simulink model "magSim3"  (Simulink 3.00)
settings: Solver=ode45  StartTime=0  StopTime=100  RelTol=1e-5
values from neighbouring files (symbols this model uses):
  Bmag = sscanf(get(findobj(gcf, 'Tag', 'EditTextBmag'),'String'), '    [CUBESIM bak.m]    (also in CUBESIM.m = sscanf(get(findobj(FIG, 'Tag', 'EditTextBmag'),'String'), '; current.mat = 1.28; current_bak.mat = 1.28; default.mat = 1.28)
  Br = 0.35    [CUBESIM bak.m]    (also in CUBESIM.m; current.mat; current_bak.mat; default.mat)
  Bs1 = sscanf(get(findobj(gcf, 'Tag', 'EditTextBs1'),'String'), '    [CUBESIM bak.m]    (also in CUBESIM.m = sscanf(get(findobj(FIG, 'Tag', 'EditTextBs1'),'String'), '; current.mat = 0.73; current_bak.mat = 0.73; default.mat = 0.73)
  Bs2 = sscanf(get(findobj(gcf, 'Tag', 'EditTextBs2'),'String'), '    [CUBESIM bak.m]    (also in CUBESIM.m = sscanf(get(findobj(FIG, 'Tag', 'EditTextBs2'),'String'), '; current.mat = 0.73; current_bak.mat = 0.73; default.mat = 0.73)
  fs = get(findobj(gcf, 'Tag', 'EditTextfs'),'UserData')    [CUBESIM bak.m]    (also in CUBESIM.m = get(findobj(FIG, 'Tag', 'EditTextfs'),'UserData'); current.mat = 0.0809149305556; current_bak.mat = 0.323659722222; default.mat = 0.161829861111)
  H0 = Isc * wb0    [CUBESIM bak.m]    (also in CUBESIM.m; current.mat = [0.00110737714815 0.0010993416399 0.00032293142175]; current_bak.mat = [-5e-05 -5e-05 0.001]; default.mat = [0 0 0.001])
  Hc = 1.59    [CUBESIM bak.m]    (also in CUBESIM.m; current.mat; current_bak.mat; default.mat = 1)
  Jinv = Isc^(-1)    [CUBESIM bak.m]    (also in CUBESIM.m; current.mat = [94.7867649385  0.000760150942758  0.106731312353; 0.0007601; current_bak.mat = [502.645502646  26.455026455  26.455026455; 26.455026455  50; default.mat = [500  0  0; 0  500  0; 0  0  500])
  q0 = [q1; q2; q3; q4]./sqrt(q1^2+q2^2+q3^2+q4^2)    [CUBESIM bak.m]    (also in CUBESIM.m; current.mat = [0 0 0 1]; current_bak.mat = [0 0 0 1]; default.mat = [0 0 0 1])
  sw = get(findobj(gcf, 'Tag', 'ButtonSW1'),'UserData')    [CUBESIM bak.m]    (also in CUBESIM.m = get(findobj(FIG, 'Tag', 'ButtonSW1'),'UserData'); current.mat = 1; current_bak.mat = 1; default.mat = 1)
  uhyst1 = [uhyst1x; uhyst1y; uhyst1z]./ norm([uhyst1x; uhyst1y; uhyst1z])    [CUBESIM bak.m]    (also in CUBESIM.m; current.mat = [0 1 0]; current_bak.mat = [0 1 0]; default.mat = [0 1 0])
  uhyst2 = [uhyst2x; uhyst2y; uhyst2z]./ norm([uhyst2x; uhyst2y; uhyst2z])    [CUBESIM bak.m]    (also in CUBESIM.m; current.mat = [1 0 0]; current_bak.mat = [1 0 0]; default.mat = [1 0 0])
  umag = [umagx; umagy ; umagz]./ norm([umagx; umagy ; umagz])    [CUBESIM bak.m]    (also in CUBESIM.m; current.mat = [0 0 1]; current_bak.mat = [0 0 1]; default.mat = [0 0 1])
  uo = 4*pi*1e-7    (= 1.25663706144e-06)    [constants.m]    (also in current.mat; current_bak.mat; default.mat)
  Vhyst1 = get(findobj(gcf, 'Tag', 'EditTextVhyst1'),'UserData')    [CUBESIM bak.m]    (also in CUBESIM.m = get(findobj(FIG, 'Tag', 'EditTextVhyst1'),'UserData'); current.mat = 1.004e-06; current_bak.mat = 1.004e-06; default.mat = 1.004e-06)
  Vhyst2 = get(findobj(gcf, 'Tag', 'EditTextVhyst2'),'UserData')    [CUBESIM bak.m]    (also in CUBESIM.m = get(findobj(FIG, 'Tag', 'EditTextVhyst2'),'UserData'); current.mat = 1.004e-06; current_bak.mat = 1.004e-06; default.mat = 1.004e-06)
  Vmag = get(findobj(gcf, 'Tag', 'EditTextVmag'),'UserData')    [CUBESIM bak.m]    (also in CUBESIM.m = get(findobj(FIG, 'Tag', 'EditTextVmag'),'UserData'); current.mat = 4.032e-06; current_bak.mat = 4.032e-06; default.mat = 4.032e-06)
undefined symbols (not defined in the file or in its folder): magnitude
libraries: simulink3 x17, simulink_extras x1
settings Model: Creator=Jean-Francois Levesque  LastModifiedBy=Chronos

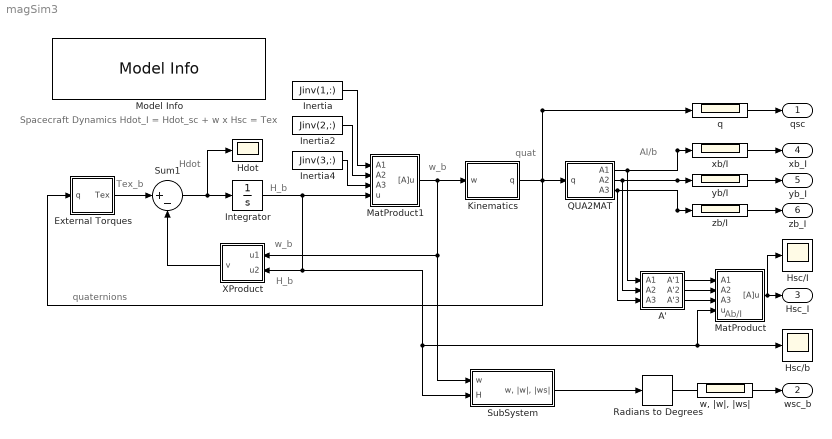
== system magSim3 ==
  note: Spacecraft Dynamics
      | Hdot_I  = Hdot_sc + w x Hsc  = Tex
  note: H_b
  note: Hdot
  note: w_b
  note: AI/b
  note: Ab/I
  note: Tex_b
  note: quat
  note: w_b
  note: H_b
  note: quaternions
  A' : Subsystem
  External Torques : Subsystem
  Hdot : Scope
      settings: TimeRange=100  YMin=-1  YMax=1  SaveToWorkspace=off  SaveName=ScopeData
  Hsc/I : Scope
      settings: TimeRange=100  YMin=-0.001  YMax=0.001  SaveToWorkspace=off  SaveName=ScopeData
  Hsc/b : Scope
      settings: TimeRange=5000  YMin=-0.0005  YMax=0.001  SaveToWorkspace=off  SaveName=ScopeData
  Inertia : Constant  Value=Jinv(1,:)
  Inertia2 : Constant  Value=Jinv(2,:)
  Inertia4 : Constant  Value=Jinv(3,:)
  Integrator : Integrator  ExternalReset=none  InitialConditionSource=internal  InitialCondition=H0  LimitOutput=off  UpperSaturationLimit=inf  LowerSaturationLimit=-inf  ShowSaturationPort=off  ShowStatePort=off  AbsoluteTolerance=auto
  Kinematics : Subsystem
  MatProduct : Subsystem
  MatProduct1 : Subsystem
  Model Info : simulink3/Signals & Systems/Model Info  InitialBlockCM=none  BlockCM=none  Frame=on  DisplayStringWithTags=|  HorizontalTextAlignment=Left  LeftAlignmentValue=0.02  SourceBlockDiagram=magSim3  TagMaxNumber=20
      | CUBESIM Attitude Dynamics
      |  Version %<ModelVersion>
      |  %<ModifiedDate>
      |  (C) 2002-2003 %<Creator>
  QUA2MAT : Subsystem
  Radians to Degrees : simulink_extras/Transformations/Radians to Degrees
  SubSystem : Subsystem
  Sum1 : Sum  Inputs=|+-  SaturateOnIntegerOverflow=on
  XProduct : Subsystem  Orientation=left
  "q " : Scope
      settings: TimeRange=100  YMin=-1  YMax=1  SaveToWorkspace=off  SaveName=ScopeData
  "w, |w|, |ws|" : Scope
      settings: TimeRange=100  YMin=-20  YMax=30  SaveToWorkspace=off  SaveName=ScopeData
  xb/I : Scope
      settings: TimeRange=100  YMin=-1  YMax=1  SaveToWorkspace=off  SaveName=ScopeData
  yb/I : Scope
      settings: TimeRange=100  YMin=-1  YMax=1  SaveToWorkspace=off  SaveName=ScopeData
  zb/I : Scope
      settings: TimeRange=100  YMin=-1  YMax=1  SaveToWorkspace=off  SaveName=ScopeData
  qsc : Outport  Port=1
  wsc_b : Outport  Port=2
  Hsc_I : Outport  Port=3
  xb_I : Outport  Port=4
  yb_I : Outport  Port=5
  zb_I : Outport  Port=6
  wires:
  External Torques/1(Tex) -> Sum1/1
  Integrator/1 -> MatProduct1/4(u), XProduct/2(u2), Hsc/b/1, MatProduct/4(u), SubSystem/2(H)
  Inertia2/1 -> MatProduct1/2(A2)
  Inertia/1 -> MatProduct1/1(A1)
  Inertia4/1 -> MatProduct1/3(A3)
  XProduct/1(v) -> Sum1/2
  Sum1/1 -> Integrator/1, Hdot/1
  MatProduct1/1("[A]u") -> Kinematics/1(w), XProduct/1(u1), SubSystem/1(w)
  Kinematics/1(q) -> QUA2MAT/1(q), qsc/1, "q "/1, External Torques/1(q)
  QUA2MAT/2(A2) -> A'/2(A2), yb/I/1, yb_I/1
  QUA2MAT/3(A3) -> A'/3(A3), zb/I/1, zb_I/1
  QUA2MAT/1(A1) -> A'/1(A1), xb/I/1, xb_I/1
  A'/1(A'1) -> MatProduct/1(A1)
  A'/2(A'2) -> MatProduct/2(A2)
  A'/3(A'3) -> MatProduct/3(A3)
  MatProduct/1("[A]u") -> Hsc_I/1, Hsc/I/1
  SubSystem/1("w, |w|, |ws|") -> Radians to Degrees/1
  Radians to Degrees/1 -> "w, |w|, |ws|"/1, wsc_b/1

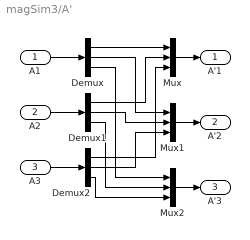
== system magSim3/A' ==
  A1 : Inport  Port=1  PortWidth=-1  SampleTime=-1  DataType=auto
      settings: SignalType=auto
  A2 : Inport  Port=2  PortWidth=-1  SampleTime=-1  DataType=auto
      settings: SignalType=auto
  A3 : Inport  Port=3  PortWidth=-1  SampleTime=-1  DataType=auto
      settings: SignalType=auto
  Demux : Demux  Outputs=3
  Demux1 : Demux  Outputs=3
  Demux2 : Demux  Outputs=3
  Mux : Mux  Inputs=3
  Mux1 : Mux  Inputs=3
  Mux2 : Mux  Inputs=3
  A'1 : Outport  Port=1
  A'2 : Outport  Port=2
  A'3 : Outport  Port=3
  wires:
  A1/1 -> Demux/1
  Demux/1 -> Mux/1
  A2/1 -> Demux1/1
  Demux1/1 -> Mux/2
  A3/1 -> Demux2/1
  Demux2/1 -> Mux/3
  Demux2/3 -> Mux2/3
  Demux1/3 -> Mux2/2
  Demux/3 -> Mux2/1
  Demux/2 -> Mux1/1
  Demux2/2 -> Mux1/3
  Demux1/2 -> Mux1/2
  Mux/1 -> A'1/1
  Mux2/1 -> A'3/1
  Mux1/1 -> A'2/1

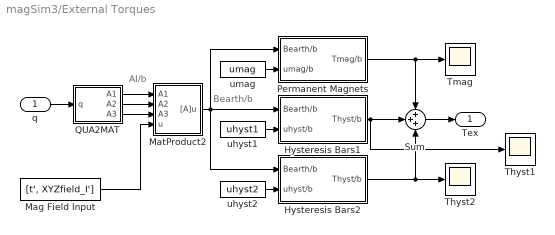
== system magSim3/External Torques ==
  note: AI/b
  note: Bearth/b
  q : Inport  Port=1  PortWidth=-1  SampleTime=-1  DataType=auto
      settings: SignalType=auto
  Hysteresis Bars1 : Subsystem
  Hysteresis Bars2 : Subsystem
  Mag Field Input : FromWorkspace  VariableName=[t', XYZfield_I']  SampleTime=1/fs  HoldFinalValue=off
  MatProduct2 : Subsystem
  Permanent Magnets : Subsystem
  QUA2MAT : Subsystem
  Sum : Sum  Inputs=+++  SaturateOnIntegerOverflow=on
  Thyst1 : Scope
      settings: TimeRange=100  YMin=-4e-005  YMax=4e-005  SaveToWorkspace=off  SaveName=ScopeData
  Thyst2 : Scope
      settings: TimeRange=100  YMin=-4e-005  YMax=4e-005  SaveToWorkspace=off  SaveName=ScopeData
  Tmag : Scope
      settings: TimeRange=100  YMin=-0.0001  YMax=0.0001  SaveToWorkspace=off  SaveName=ScopeData
  uhyst1 : Constant  Value=uhyst1
  uhyst2 : Constant  Value=uhyst2
  umag : Constant  Value=umag
  Tex : Outport  Port=1
  wires:
  umag/1 -> Permanent Magnets/2(umag/b)
  uhyst1/1 -> Hysteresis Bars1/2(uhyst/b)
  uhyst2/1 -> Hysteresis Bars2/2(uhyst/b)
  QUA2MAT/1(A1) -> MatProduct2/1(A1)
  QUA2MAT/2(A2) -> MatProduct2/2(A2)
  QUA2MAT/3(A3) -> MatProduct2/3(A3)
  MatProduct2/1("[A]u") -> Hysteresis Bars1/1(Bearth/b), Permanent Magnets/1(Bearth/b), Hysteresis Bars2/1(Bearth/b)
  Sum/1 -> Tex/1
  q/1 -> QUA2MAT/1(q)
  Permanent Magnets/1(Tmag/b) -> Tmag/1, Sum/1
  Hysteresis Bars2/1(Thyst/b) -> Thyst2/1, Sum/3
  Hysteresis Bars1/1(Thyst/b) -> Thyst1/1, Sum/2
  Mag Field Input/1 -> MatProduct2/4(u)

== system magSim3/Kinematics ==
  note: q
  note: qdot
  note: q^
  w : Inport  Port=1  PortWidth=-1  SampleTime=-1  DataType=auto
      settings: SignalType=auto
  Dot Product{,1..3} (4 alike) : simulink3/Math/Dot Product
  Gain : Gain  Gain=1/2  SaturateOnIntegerOverflow=on
  Integrator : Integrator  ExternalReset=none  InitialConditionSource=internal  InitialCondition=q0  LimitOutput=off  UpperSaturationLimit=inf  LowerSaturationLimit=-inf  ShowSaturationPort=off  ShowStatePort=off  AbsoluteTolerance=auto
  Mux2 : Mux  Inputs=4
  Omega : Subsystem
  Product : Product  Inputs=*/  SaturateOnIntegerOverflow=on
  VecNorm : Subsystem
  q : Outport  Port=1
  wires:
  Dot Product/1 -> Mux2/1
  Dot Product1/1 -> Mux2/2
  Dot Product2/1 -> Mux2/3
  Dot Product3/1 -> Mux2/4
  Gain/1 -> Integrator/1
  Mux2/1 -> Gain/1
  VecNorm/1(|u|) -> Product/2
  Integrator/1 -> Product/1, VecNorm/1(u), Dot Product2/2, Dot Product1/2, Dot Product/2, Dot Product3/2
  Omega/1(Omega1) -> Dot Product/1
  Omega/2(Omega2) -> Dot Product1/1
  Omega/3(Omega3) -> Dot Product2/1
  Omega/4(Omega4) -> Dot Product3/1
  Product/1 -> q/1
  w/1 -> Omega/1(w)

== system magSim3/MatProduct ==
  A1 : Inport  Port=1  PortWidth=-1  SampleTime=-1  DataType=auto
      settings: SignalType=auto
  A2 : Inport  Port=2  PortWidth=-1  SampleTime=-1  DataType=auto
      settings: SignalType=auto
  A3 : Inport  Port=3  PortWidth=-1  SampleTime=-1  DataType=auto
      settings: SignalType=auto
  u : Inport  Port=4  PortWidth=-1  SampleTime=-1  DataType=auto
      settings: SignalType=auto
  Dot Product4 : simulink3/Math/Dot Product
  Dot Product5 : simulink3/Math/Dot Product
  Dot Product6 : simulink3/Math/Dot Product
  Mux2 : Mux  Inputs=3
  "[A]u" : Outport  Port=1
  wires:
  Dot Product4/1 -> Mux2/1
  Dot Product5/1 -> Mux2/2
  Dot Product6/1 -> Mux2/3
  A1/1 -> Dot Product4/1
  Mux2/1 -> "[A]u"/1
  A2/1 -> Dot Product5/1
  A3/1 -> Dot Product6/1
  u/1 -> Dot Product6/2, Dot Product4/2, Dot Product5/2

== system magSim3/MatProduct1 ==
  A1 : Inport  Port=1  PortWidth=-1  SampleTime=-1  DataType=auto
      settings: SignalType=auto
  A2 : Inport  Port=2  PortWidth=-1  SampleTime=-1  DataType=auto
      settings: SignalType=auto
  A3 : Inport  Port=3  PortWidth=-1  SampleTime=-1  DataType=auto
      settings: SignalType=auto
  u : Inport  Port=4  PortWidth=-1  SampleTime=-1  DataType=auto
      settings: SignalType=auto
  Dot Product4 : simulink3/Math/Dot Product
  Dot Product5 : simulink3/Math/Dot Product
  Dot Product6 : simulink3/Math/Dot Product
  Mux2 : Mux  Inputs=3
  "[A]u" : Outport  Port=1
  wires:
  Dot Product4/1 -> Mux2/1
  Dot Product5/1 -> Mux2/2
  Dot Product6/1 -> Mux2/3
  A1/1 -> Dot Product4/1
  Mux2/1 -> "[A]u"/1
  A2/1 -> Dot Product5/1
  A3/1 -> Dot Product6/1
  u/1 -> Dot Product6/2, Dot Product4/2, Dot Product5/2

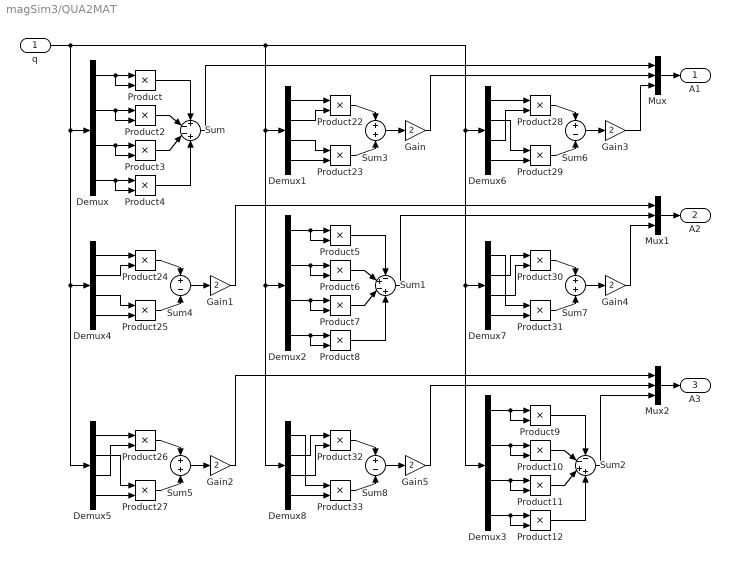
== system magSim3/QUA2MAT ==
  q : Inport  Port=1  PortWidth=-1  SampleTime=-1  DataType=auto
      settings: SignalType=auto
  Demux{,1..8} (9 alike) : Demux  Outputs=4
  Gain{,1..5} (6 alike) : Gain  Gain=2  SaturateOnIntegerOverflow=on
  Mux : Mux  Inputs=3
  Mux1 : Mux  Inputs=3
  Mux2 : Mux  Inputs=3
  Product{,2..12,22..33} (24 alike) : Product  Inputs=2  SaturateOnIntegerOverflow=on
  Sum : Sum  Inputs=+--+  SaturateOnIntegerOverflow=on
  Sum1 : Sum  Inputs=-+-+  SaturateOnIntegerOverflow=on
  Sum2 : Sum  Inputs=--++  SaturateOnIntegerOverflow=on
  Sum3 : Sum  Inputs=++  SaturateOnIntegerOverflow=on
  Sum4 : Sum  Inputs=+-  SaturateOnIntegerOverflow=on
  Sum5 : Sum  Inputs=++  SaturateOnIntegerOverflow=on
  Sum6 : Sum  Inputs=+-  SaturateOnIntegerOverflow=on
  Sum7 : Sum  Inputs=++  SaturateOnIntegerOverflow=on
  Sum8 : Sum  Inputs=+-  SaturateOnIntegerOverflow=on
  A1 : Outport  Port=1
  A2 : Outport  Port=2
  A3 : Outport  Port=3
  wires:
  Demux/1 -> Product/1, Product/2
  Demux/2 -> Product2/1, Product2/2
  Demux/3 -> Product3/1, Product3/2
  Demux/4 -> Product4/1, Product4/2
  Product/1 -> Sum/1
  Product4/1 -> Sum/4
  Product3/1 -> Sum/3
  Product2/1 -> Sum/2
  Product23/1 -> Sum3/2
  Demux1/1 -> Product22/1
  Demux1/4 -> Product23/2
  Demux1/3 -> Product23/1
  Demux1/2 -> Product22/2
  Sum3/1 -> Gain/1
  Product22/1 -> Sum3/1
  Product29/1 -> Sum6/2
  Demux6/1 -> Product28/1
  Demux6/4 -> Product29/2
  Sum6/1 -> Gain3/1
  Product28/1 -> Sum6/1
  q/1 -> Demux3/1, Demux7/1, Demux6/1, Demux1/1, Demux8/1, Demux2/1, Demux/1, Demux5/1, Demux4/1
  Demux6/3 -> Product28/2
  Demux6/2 -> Product29/1
  Product25/1 -> Sum4/2
  Demux4/1 -> Product24/1
  Demux4/4 -> Product25/2
  Demux4/3 -> Product25/1
  Demux4/2 -> Product24/2
  Sum4/1 -> Gain1/1
  Product24/1 -> Sum4/1
  Demux2/1 -> Product5/1, Product5/2
  Demux2/2 -> Product6/1, Product6/2
  Demux2/3 -> Product7/1, Product7/2
  Demux2/4 -> Product8/1, Product8/2
  Product5/1 -> Sum1/1
  Product8/1 -> Sum1/4
  Product7/1 -> Sum1/3
  Product6/1 -> Sum1/2
  Product31/1 -> Sum7/2
  Demux7/4 -> Product31/2
  Sum7/1 -> Gain4/1
  Product30/1 -> Sum7/1
  Demux7/1 -> Product31/1
  Demux7/2 -> Product30/1
  Demux7/3 -> Product30/2
  Product27/1 -> Sum5/2
  Demux5/1 -> Product26/1
  Demux5/4 -> Product27/2
  Sum5/1 -> Gain2/1
  Product26/1 -> Sum5/1
  Product33/1 -> Sum8/2
  Demux8/4 -> Product33/2
  Sum8/1 -> Gain5/1
  Product32/1 -> Sum8/1
  Demux3/1 -> Product9/1, Product9/2
  Demux3/2 -> Product10/1, Product10/2
  Demux3/3 -> Product11/1, Product11/2
  Demux3/4 -> Product12/1, Product12/2
  Product9/1 -> Sum2/1
  Product12/1 -> Sum2/4
  Product11/1 -> Sum2/3
  Product10/1 -> Sum2/2
  Demux5/3 -> Product26/2
  Demux5/2 -> Product27/1
  Demux8/2 -> Product32/1
  Demux8/3 -> Product32/2
  Demux8/1 -> Product33/1
  Sum1/1 -> Mux1/2
  Mux1/1 -> A2/1
  Gain/1 -> Mux/2
  Mux/1 -> A1/1
  Gain3/1 -> Mux/3
  Sum/1 -> Mux/1
  Gain1/1 -> Mux1/1
  Gain4/1 -> Mux1/3
  Gain5/1 -> Mux2/2
  Mux2/1 -> A3/1
  Gain2/1 -> Mux2/1
  Sum2/1 -> Mux2/3

== system magSim3/SubSystem ==
  note: H^
  note: w
  note: |w|
  note: |ws|
  w : Inport  Port=1  PortWidth=-1  SampleTime=-1  DataType=auto
      settings: SignalType=auto
  H : Inport  Port=2  PortWidth=-1  SampleTime=-1  DataType=auto
      settings: SignalType=auto
  Dot Product3 : simulink3/Math/Dot Product
  Mux1 : Mux  Inputs=3
  Product : Product  Inputs=*/  SaturateOnIntegerOverflow=on
  VecNorm : Subsystem
  VecNorm1 : Subsystem
  "w, |w|, |ws|" : Outport  Port=1
  wires:
  VecNorm1/1(|u|) -> Mux1/2
  Dot Product3/1 -> Mux1/3
  VecNorm/1(|u|) -> Product/2
  Product/1 -> Dot Product3/2
  w/1 -> Dot Product3/1, Mux1/1, VecNorm1/1(u)
  H/1 -> VecNorm/1(u), Product/1
  Mux1/1 -> "w, |w|, |ws|"/1

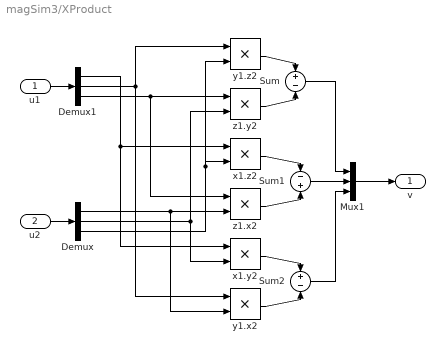
== system magSim3/XProduct ==
  u1 : Inport  Port=1  PortWidth=-1  SampleTime=-1  DataType=auto
      settings: SignalType=auto
  u2 : Inport  Port=2  PortWidth=-1  SampleTime=-1  DataType=auto
      settings: SignalType=auto
  Demux : Demux  Outputs=3
  Demux1 : Demux  Outputs=3
  Mux1 : Mux  Inputs=3
  Sum : Sum  Inputs=+-  SaturateOnIntegerOverflow=on
  Sum1 : Sum  Inputs=-+  SaturateOnIntegerOverflow=on
  Sum2 : Sum  Inputs=+-  SaturateOnIntegerOverflow=on
  x1.y2 : Product  Inputs=2  SaturateOnIntegerOverflow=on
  x1.z2 : Product  Inputs=2  SaturateOnIntegerOverflow=on
  y1.x2 : Product  Inputs=2  SaturateOnIntegerOverflow=on
  y1.z2 : Product  Inputs=2  SaturateOnIntegerOverflow=on
  z1.x2 : Product  Inputs=2  SaturateOnIntegerOverflow=on
  z1.y2 : Product  Inputs=2  SaturateOnIntegerOverflow=on
  v : Outport  Port=1
  wires:
  u1/1 -> Demux1/1
  Demux1/2 -> y1.z2/1, y1.x2/1
  Demux1/1 -> x1.y2/1, x1.z2/1
  Demux1/3 -> z1.x2/1, z1.y2/1
  y1.z2/1 -> Sum/1
  z1.y2/1 -> Sum/2
  x1.z2/1 -> Sum1/1
  z1.x2/1 -> Sum1/2
  x1.y2/1 -> Sum2/1
  y1.x2/1 -> Sum2/2
  Sum1/1 -> Mux1/2
  Sum/1 -> Mux1/1
  Sum2/1 -> Mux1/3
  Mux1/1 -> v/1
  Demux/3 -> y1.z2/2, x1.z2/2
  Demux/2 -> x1.y2/2, z1.y2/2
  Demux/1 -> z1.x2/2, y1.x2/2
  u2/1 -> Demux/1

== system magSim3/External Torques/Hysteresis Bars1 ==
  note: m x B
  Bearth/b : Inport  Port=1  PortWidth=-1  SampleTime=-1  DataType=auto
      settings: SignalType=auto
  uhyst/b : Inport  Port=2  PortWidth=-1  SampleTime=-1  DataType=auto
      settings: SignalType=auto
  Hysteresis Model : Subsystem
  XProduct : Subsystem
  Thyst/b : Outport  Port=1
  wires:
  Hysteresis Model/1(mhyst) -> XProduct/1(u1)
  uhyst/b/1 -> Hysteresis Model/1(uhyst)
  XProduct/1(v) -> Thyst/b/1
  Bearth/b/1 -> XProduct/2(u2), Hysteresis Model/2(Bearth/b)

== system magSim3/External Torques/Hysteresis Bars2 ==
  note: m x B
  Bearth/b : Inport  Port=1  PortWidth=-1  SampleTime=-1  DataType=auto
      settings: SignalType=auto
  uhyst/b : Inport  Port=2  PortWidth=-1  SampleTime=-1  DataType=auto
      settings: SignalType=auto
  Hysteresis Model : Subsystem
  XProduct : Subsystem
  Thyst/b : Outport  Port=1
  wires:
  XProduct/1(v) -> Thyst/b/1
  Bearth/b/1 -> XProduct/2(u2), Hysteresis Model/2(Bearth/b)
  uhyst/b/1 -> Hysteresis Model/1(uhyst)
  Hysteresis Model/1(mhyst) -> XProduct/1(u1)

== system magSim3/External Torques/MatProduct2 ==
  A1 : Inport  Port=1  PortWidth=-1  SampleTime=-1  DataType=auto
      settings: SignalType=auto
  A2 : Inport  Port=2  PortWidth=-1  SampleTime=-1  DataType=auto
      settings: SignalType=auto
  A3 : Inport  Port=3  PortWidth=-1  SampleTime=-1  DataType=auto
      settings: SignalType=auto
  u : Inport  Port=4  PortWidth=-1  SampleTime=-1  DataType=auto
      settings: SignalType=auto
  Dot Product4 : simulink3/Math/Dot Product
  Dot Product5 : simulink3/Math/Dot Product
  Dot Product6 : simulink3/Math/Dot Product
  Mux2 : Mux  Inputs=3
  "[A]u" : Outport  Port=1
  wires:
  Dot Product4/1 -> Mux2/1
  Dot Product5/1 -> Mux2/2
  Dot Product6/1 -> Mux2/3
  A1/1 -> Dot Product4/1
  Mux2/1 -> "[A]u"/1
  A2/1 -> Dot Product5/1
  A3/1 -> Dot Product6/1
  u/1 -> Dot Product6/2, Dot Product4/2, Dot Product5/2

== system magSim3/External Torques/Permanent Magnets ==
  note: m x B
  note: mmag
  Bearth/b : Inport  Port=1  PortWidth=-1  SampleTime=-1  DataType=auto
      settings: SignalType=auto
  umag/b : Inport  Port=2  PortWidth=-1  SampleTime=-1  DataType=auto
      settings: SignalType=auto
  Bmag : Constant  Value=Bmag
  Product : Product  Inputs=2  SaturateOnIntegerOverflow=on
  Vmag/uo : Gain  Gain=Vmag/uo  SaturateOnIntegerOverflow=on
  XProduct : Subsystem
  Tmag/b : Outport  Port=1
  wires:
  Bearth/b/1 -> XProduct/2(u2)
  Bmag/1 -> Vmag/uo/1
  Vmag/uo/1 -> Product/2
  umag/b/1 -> Product/1
  Product/1 -> XProduct/1(u1)
  XProduct/1(v) -> Tmag/b/1

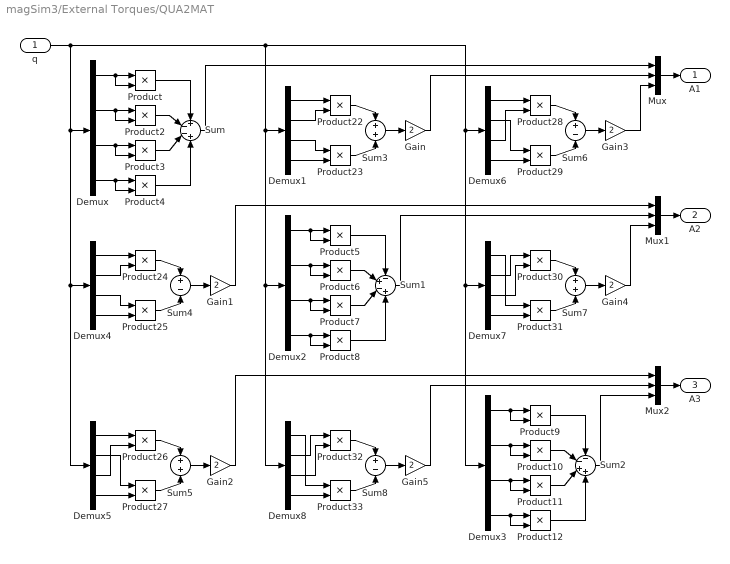
== system magSim3/External Torques/QUA2MAT ==
  q : Inport  Port=1  PortWidth=-1  SampleTime=-1  DataType=auto
      settings: SignalType=auto
  Demux{,1..8} (9 alike) : Demux  Outputs=4
  Gain{,1..5} (6 alike) : Gain  Gain=2  SaturateOnIntegerOverflow=on
  Mux : Mux  Inputs=3
  Mux1 : Mux  Inputs=3
  Mux2 : Mux  Inputs=3
  Product{,2..12,22..33} (24 alike) : Product  Inputs=2  SaturateOnIntegerOverflow=on
  Sum : Sum  Inputs=+--+  SaturateOnIntegerOverflow=on
  Sum1 : Sum  Inputs=-+-+  SaturateOnIntegerOverflow=on
  Sum2 : Sum  Inputs=--++  SaturateOnIntegerOverflow=on
  Sum3 : Sum  Inputs=++  SaturateOnIntegerOverflow=on
  Sum4 : Sum  Inputs=+-  SaturateOnIntegerOverflow=on
  Sum5 : Sum  Inputs=++  SaturateOnIntegerOverflow=on
  Sum6 : Sum  Inputs=+-  SaturateOnIntegerOverflow=on
  Sum7 : Sum  Inputs=++  SaturateOnIntegerOverflow=on
  Sum8 : Sum  Inputs=+-  SaturateOnIntegerOverflow=on
  A1 : Outport  Port=1
  A2 : Outport  Port=2
  A3 : Outport  Port=3
  wires:
  Demux/1 -> Product/1, Product/2
  Demux/2 -> Product2/1, Product2/2
  Demux/3 -> Product3/1, Product3/2
  Demux/4 -> Product4/1, Product4/2
  Product/1 -> Sum/1
  Product4/1 -> Sum/4
  Product3/1 -> Sum/3
  Product2/1 -> Sum/2
  Product23/1 -> Sum3/2
  Demux1/1 -> Product22/1
  Demux1/4 -> Product23/2
  Demux1/3 -> Product23/1
  Demux1/2 -> Product22/2
  Sum3/1 -> Gain/1
  Product22/1 -> Sum3/1
  Product29/1 -> Sum6/2
  Demux6/1 -> Product28/1
  Demux6/4 -> Product29/2
  Sum6/1 -> Gain3/1
  Product28/1 -> Sum6/1
  q/1 -> Demux3/1, Demux7/1, Demux6/1, Demux1/1, Demux8/1, Demux2/1, Demux/1, Demux5/1, Demux4/1
  Demux6/3 -> Product28/2
  Demux6/2 -> Product29/1
  Product25/1 -> Sum4/2
  Demux4/1 -> Product24/1
  Demux4/4 -> Product25/2
  Demux4/3 -> Product25/1
  Demux4/2 -> Product24/2
  Sum4/1 -> Gain1/1
  Product24/1 -> Sum4/1
  Demux2/1 -> Product5/1, Product5/2
  Demux2/2 -> Product6/1, Product6/2
  Demux2/3 -> Product7/1, Product7/2
  Demux2/4 -> Product8/1, Product8/2
  Product5/1 -> Sum1/1
  Product8/1 -> Sum1/4
  Product7/1 -> Sum1/3
  Product6/1 -> Sum1/2
  Product31/1 -> Sum7/2
  Demux7/4 -> Product31/2
  Sum7/1 -> Gain4/1
  Product30/1 -> Sum7/1
  Demux7/1 -> Product31/1
  Demux7/2 -> Product30/1
  Demux7/3 -> Product30/2
  Product27/1 -> Sum5/2
  Demux5/1 -> Product26/1
  Demux5/4 -> Product27/2
  Sum5/1 -> Gain2/1
  Product26/1 -> Sum5/1
  Product33/1 -> Sum8/2
  Demux8/4 -> Product33/2
  Sum8/1 -> Gain5/1
  Product32/1 -> Sum8/1
  Demux3/1 -> Product9/1, Product9/2
  Demux3/2 -> Product10/1, Product10/2
  Demux3/3 -> Product11/1, Product11/2
  Demux3/4 -> Product12/1, Product12/2
  Product9/1 -> Sum2/1
  Product12/1 -> Sum2/4
  Product11/1 -> Sum2/3
  Product10/1 -> Sum2/2
  Demux5/3 -> Product26/2
  Demux5/2 -> Product27/1
  Demux8/2 -> Product32/1
  Demux8/3 -> Product32/2
  Demux8/1 -> Product33/1
  Sum1/1 -> Mux1/2
  Mux1/1 -> A2/1
  Gain/1 -> Mux/2
  Mux/1 -> A1/1
  Gain3/1 -> Mux/3
  Sum/1 -> Mux/1
  Gain1/1 -> Mux1/1
  Gain4/1 -> Mux1/3
  Gain5/1 -> Mux2/2
  Mux2/1 -> A3/1
  Gain2/1 -> Mux2/1
  Sum2/1 -> Mux2/3

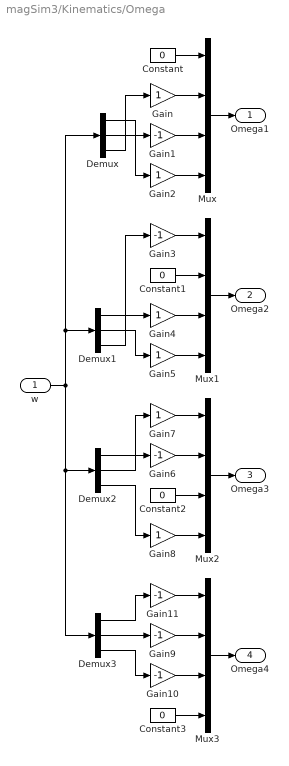
== system magSim3/Kinematics/Omega ==
  w : Inport  Port=1  PortWidth=-1  SampleTime=-1  DataType=auto
      settings: SignalType=auto
  Constant{,1..3} (4 alike) : Constant  Value=0
  Demux{,1..3} (4 alike) : Demux  Outputs=3
  Gain{,2,4..5,7..8} (6 alike) : Gain  Gain=1  SaturateOnIntegerOverflow=on
  Gain{1,3,6,9..11} (6 alike) : Gain  Gain=-1  SaturateOnIntegerOverflow=on
  Mux{,1..3} (4 alike) : Mux  Inputs=4
  Omega1 : Outport  Port=1
  Omega2 : Outport  Port=2
  Omega3 : Outport  Port=3
  Omega4 : Outport  Port=4
  wires:
  Gain/1 -> Mux/2
  Gain1/1 -> Mux/3
  Gain2/1 -> Mux/4
  Constant/1 -> Mux/1
  Gain4/1 -> Mux1/3
  Gain5/1 -> Mux1/4
  Gain6/1 -> Mux2/2
  Gain8/1 -> Mux2/4
  Gain9/1 -> Mux3/2
  Gain10/1 -> Mux3/3
  Gain3/1 -> Mux1/1
  Constant1/1 -> Mux1/2
  Gain7/1 -> Mux2/1
  Constant2/1 -> Mux2/3
  Gain11/1 -> Mux3/1
  Constant3/1 -> Mux3/4
  Demux/1 -> Gain2/1
  Demux/2 -> Gain1/1
  Demux/3 -> Gain/1
  Demux1/3 -> Gain3/1
  Demux1/1 -> Gain4/1
  Demux1/2 -> Gain5/1
  Demux2/1 -> Gain6/1
  Demux2/2 -> Gain7/1
  Demux2/3 -> Gain8/1
  Demux3/1 -> Gain11/1
  Demux3/2 -> Gain9/1
  Demux3/3 -> Gain10/1
  w/1 -> Demux/1, Demux1/1, Demux3/1, Demux2/1
  Mux1/1 -> Omega2/1
  Mux3/1 -> Omega4/1
  Mux2/1 -> Omega3/1
  Mux/1 -> Omega1/1

== system magSim3/Kinematics/VecNorm ==
  u : Inport  Port=1  PortWidth=-1  SampleTime=-1  DataType=auto
      settings: SignalType=auto
  Math Function : Math  Operator=magnitude^2  OutputSignalType=auto
  Math Function1 : Math  Operator=sqrt  OutputSignalType=auto
  Sum : Sum  Inputs=1  SaturateOnIntegerOverflow=on
  |u| : Outport  Port=1
  wires:
  Sum/1 -> Math Function1/1
  Math Function/1 -> Sum/1
  u/1 -> Math Function/1
  Math Function1/1 -> |u|/1

== system magSim3/SubSystem/VecNorm ==
  u : Inport  Port=1  PortWidth=-1  SampleTime=-1  DataType=auto
      settings: SignalType=auto
  Math Function : Math  Operator=magnitude^2  OutputSignalType=auto
  Math Function1 : Math  Operator=sqrt  OutputSignalType=auto
  Sum : Sum  Inputs=1  SaturateOnIntegerOverflow=on
  |u| : Outport  Port=1
  wires:
  Sum/1 -> Math Function1/1
  Math Function/1 -> Sum/1
  u/1 -> Math Function/1
  Math Function1/1 -> |u|/1

== system magSim3/SubSystem/VecNorm1 ==
  u : Inport  Port=1  PortWidth=-1  SampleTime=-1  DataType=auto
      settings: SignalType=auto
  Math Function : Math  Operator=magnitude^2  OutputSignalType=auto
  Math Function1 : Math  Operator=sqrt  OutputSignalType=auto
  Sum : Sum  Inputs=1  SaturateOnIntegerOverflow=on
  |u| : Outport  Port=1
  wires:
  Sum/1 -> Math Function1/1
  Math Function/1 -> Sum/1
  u/1 -> Math Function/1
  Math Function1/1 -> |u|/1

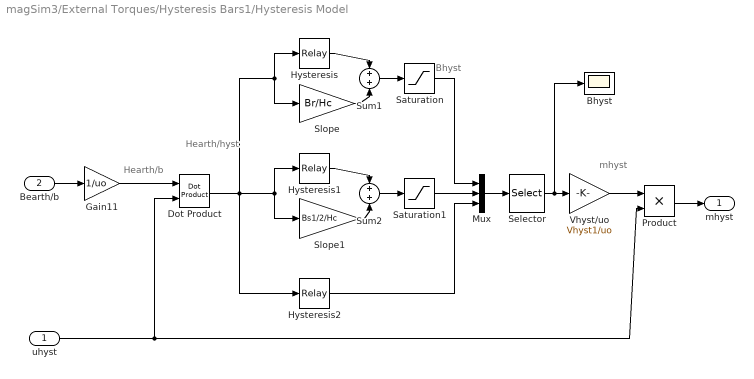
== system magSim3/External Torques/Hysteresis Bars1/Hysteresis Model ==
  note: Bhyst
  note: Hearth/b
  note: Hearth/hyst
  note: mhyst
  uhyst : Inport  Port=1  PortWidth=-1  SampleTime=-1  DataType=auto
      settings: SignalType=auto
  Bearth/b : Inport  Port=2  PortWidth=-1  SampleTime=-1  DataType=auto
      settings: SignalType=auto
  Bhyst : Scope
      settings: TimeRange=100  YMin=-1  YMax=1  SaveToWorkspace=off  SaveName=ScopeData
  Dot Product : simulink3/Math/Dot Product
  Gain11 : Gain  Gain=1/uo  SaturateOnIntegerOverflow=on
  Hysteresis : Relay  OnSwitchValue=Hc  OffSwitchValue=-Hc  OnOutputValue=Br  OffOutputValue=-Br
  Hysteresis1 : Relay  OnSwitchValue=Hc  OffSwitchValue=-Hc  OnOutputValue=Br  OffOutputValue=-Br
  Hysteresis2 : Relay  OnSwitchValue=Hc  OffSwitchValue=-Hc  OnOutputValue=Bs1  OffOutputValue=-Bs1
  Mux : Mux  Inputs=3
  Product : Product  Inputs=2  SaturateOnIntegerOverflow=on
  Saturation : Saturate  UpperLimit=Bs1  LowerLimit=-Bs1
  Saturation1 : Saturate  UpperLimit=Bs1  LowerLimit=-Bs1
  Selector : Selector  Elements=[sw]  InputPortWidth=3
  Slope : Gain  Gain=Br/Hc  SaturateOnIntegerOverflow=on
  Slope1 : Gain  Gain=Bs1/2/Hc  SaturateOnIntegerOverflow=on
  Sum1 : Sum  Inputs=+|+  SaturateOnIntegerOverflow=on
  Sum2 : Sum  Inputs=+|+  SaturateOnIntegerOverflow=on
  Vhyst/uo : Gain  Gain=Vhyst1/uo  SaturateOnIntegerOverflow=on
  mhyst : Outport  Port=1
  wires:
  Slope/1 -> Sum1/2
  Hysteresis/1 -> Sum1/1
  Sum1/1 -> Saturation/1
  uhyst/1 -> Dot Product/2, Product/2
  Slope1/1 -> Sum2/2
  Hysteresis1/1 -> Sum2/1
  Sum2/1 -> Saturation1/1
  Mux/1 -> Selector/1
  Saturation1/1 -> Mux/2
  Saturation/1 -> Mux/1
  Product/1 -> mhyst/1
  Vhyst/uo/1 -> Product/1
  Dot Product/1 -> Hysteresis2/1, Slope1/1, Hysteresis1/1, Slope/1, Hysteresis/1
  Bearth/b/1 -> Gain11/1
  Gain11/1 -> Dot Product/1
  Hysteresis2/1 -> Mux/3
  Selector/1 -> Vhyst/uo/1, Bhyst/1

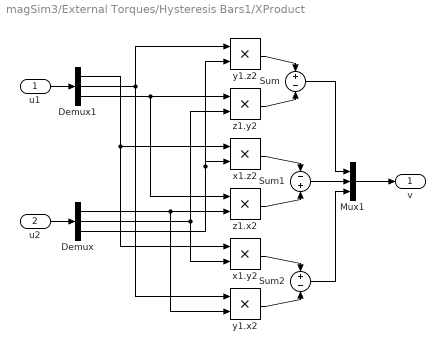
== system magSim3/External Torques/Hysteresis Bars1/XProduct ==
  u1 : Inport  Port=1  PortWidth=-1  SampleTime=-1  DataType=auto
      settings: SignalType=auto
  u2 : Inport  Port=2  PortWidth=-1  SampleTime=-1  DataType=auto
      settings: SignalType=auto
  Demux : Demux  Outputs=3
  Demux1 : Demux  Outputs=3
  Mux1 : Mux  Inputs=3
  Sum : Sum  Inputs=+-  SaturateOnIntegerOverflow=on
  Sum1 : Sum  Inputs=-+  SaturateOnIntegerOverflow=on
  Sum2 : Sum  Inputs=+-  SaturateOnIntegerOverflow=on
  x1.y2 : Product  Inputs=2  SaturateOnIntegerOverflow=on
  x1.z2 : Product  Inputs=2  SaturateOnIntegerOverflow=on
  y1.x2 : Product  Inputs=2  SaturateOnIntegerOverflow=on
  y1.z2 : Product  Inputs=2  SaturateOnIntegerOverflow=on
  z1.x2 : Product  Inputs=2  SaturateOnIntegerOverflow=on
  z1.y2 : Product  Inputs=2  SaturateOnIntegerOverflow=on
  v : Outport  Port=1
  wires:
  u1/1 -> Demux1/1
  Demux1/2 -> y1.z2/1, y1.x2/1
  Demux1/1 -> x1.y2/1, x1.z2/1
  Demux1/3 -> z1.x2/1, z1.y2/1
  y1.z2/1 -> Sum/1
  z1.y2/1 -> Sum/2
  x1.z2/1 -> Sum1/1
  z1.x2/1 -> Sum1/2
  x1.y2/1 -> Sum2/1
  y1.x2/1 -> Sum2/2
  Sum1/1 -> Mux1/2
  Sum/1 -> Mux1/1
  Sum2/1 -> Mux1/3
  Mux1/1 -> v/1
  Demux/3 -> y1.z2/2, x1.z2/2
  Demux/2 -> x1.y2/2, z1.y2/2
  Demux/1 -> z1.x2/2, y1.x2/2
  u2/1 -> Demux/1

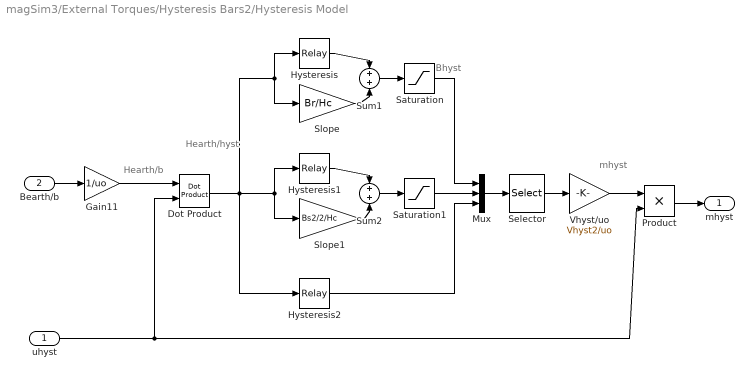
== system magSim3/External Torques/Hysteresis Bars2/Hysteresis Model ==
  note: Bhyst
  note: Hearth/b
  note: Hearth/hyst
  note: mhyst
  uhyst : Inport  Port=1  PortWidth=-1  SampleTime=-1  DataType=auto
      settings: SignalType=auto
  Bearth/b : Inport  Port=2  PortWidth=-1  SampleTime=-1  DataType=auto
      settings: SignalType=auto
  Dot Product : simulink3/Math/Dot Product
  Gain11 : Gain  Gain=1/uo  SaturateOnIntegerOverflow=on
  Hysteresis : Relay  OnSwitchValue=Hc  OffSwitchValue=-Hc  OnOutputValue=Br  OffOutputValue=-Br
  Hysteresis1 : Relay  OnSwitchValue=Hc  OffSwitchValue=-Hc  OnOutputValue=Br  OffOutputValue=-Br
  Hysteresis2 : Relay  OnSwitchValue=Hc  OffSwitchValue=-Hc  OnOutputValue=Bs2  OffOutputValue=-Bs2
  Mux : Mux  Inputs=3
  Product : Product  Inputs=2  SaturateOnIntegerOverflow=on
  Saturation : Saturate  UpperLimit=Bs2  LowerLimit=-Bs2
  Saturation1 : Saturate  UpperLimit=Bs2  LowerLimit=-Bs2
  Selector : Selector  Elements=[sw]  InputPortWidth=3
  Slope : Gain  Gain=Br/Hc  SaturateOnIntegerOverflow=on
  Slope1 : Gain  Gain=Bs2/2/Hc  SaturateOnIntegerOverflow=on
  Sum1 : Sum  Inputs=+|+  SaturateOnIntegerOverflow=on
  Sum2 : Sum  Inputs=+|+  SaturateOnIntegerOverflow=on
  Vhyst/uo : Gain  Gain=Vhyst2/uo  SaturateOnIntegerOverflow=on
  mhyst : Outport  Port=1
  wires:
  Slope/1 -> Sum1/2
  Hysteresis/1 -> Sum1/1
  Sum1/1 -> Saturation/1
  uhyst/1 -> Dot Product/2, Product/2
  Slope1/1 -> Sum2/2
  Hysteresis1/1 -> Sum2/1
  Sum2/1 -> Saturation1/1
  Mux/1 -> Selector/1
  Saturation1/1 -> Mux/2
  Hysteresis2/1 -> Mux/3
  Saturation/1 -> Mux/1
  Selector/1 -> Vhyst/uo/1
  Product/1 -> mhyst/1
  Dot Product/1 -> Hysteresis2/1, Slope1/1, Hysteresis1/1, Slope/1, Hysteresis/1
  Bearth/b/1 -> Gain11/1
  Gain11/1 -> Dot Product/1
  Vhyst/uo/1 -> Product/1

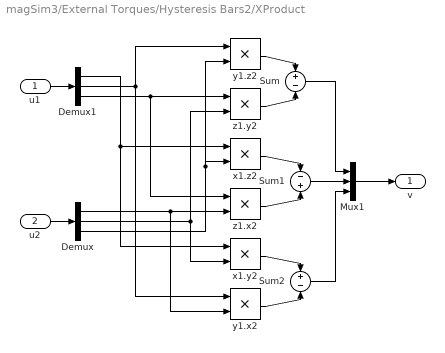
== system magSim3/External Torques/Hysteresis Bars2/XProduct ==
  u1 : Inport  Port=1  PortWidth=-1  SampleTime=-1  DataType=auto
      settings: SignalType=auto
  u2 : Inport  Port=2  PortWidth=-1  SampleTime=-1  DataType=auto
      settings: SignalType=auto
  Demux : Demux  Outputs=3
  Demux1 : Demux  Outputs=3
  Mux1 : Mux  Inputs=3
  Sum : Sum  Inputs=+-  SaturateOnIntegerOverflow=on
  Sum1 : Sum  Inputs=-+  SaturateOnIntegerOverflow=on
  Sum2 : Sum  Inputs=+-  SaturateOnIntegerOverflow=on
  x1.y2 : Product  Inputs=2  SaturateOnIntegerOverflow=on
  x1.z2 : Product  Inputs=2  SaturateOnIntegerOverflow=on
  y1.x2 : Product  Inputs=2  SaturateOnIntegerOverflow=on
  y1.z2 : Product  Inputs=2  SaturateOnIntegerOverflow=on
  z1.x2 : Product  Inputs=2  SaturateOnIntegerOverflow=on
  z1.y2 : Product  Inputs=2  SaturateOnIntegerOverflow=on
  v : Outport  Port=1
  wires:
  u1/1 -> Demux1/1
  Demux1/2 -> y1.z2/1, y1.x2/1
  Demux1/1 -> x1.y2/1, x1.z2/1
  Demux1/3 -> z1.x2/1, z1.y2/1
  y1.z2/1 -> Sum/1
  z1.y2/1 -> Sum/2
  x1.z2/1 -> Sum1/1
  z1.x2/1 -> Sum1/2
  x1.y2/1 -> Sum2/1
  y1.x2/1 -> Sum2/2
  Sum1/1 -> Mux1/2
  Sum/1 -> Mux1/1
  Sum2/1 -> Mux1/3
  Mux1/1 -> v/1
  Demux/3 -> y1.z2/2, x1.z2/2
  Demux/2 -> x1.y2/2, z1.y2/2
  Demux/1 -> z1.x2/2, y1.x2/2
  u2/1 -> Demux/1

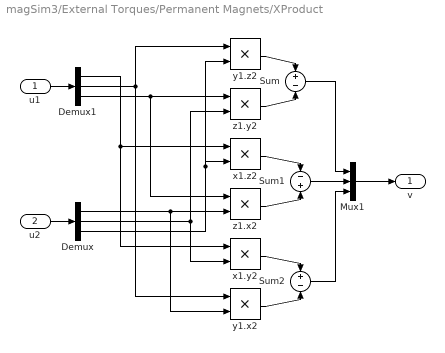
== system magSim3/External Torques/Permanent Magnets/XProduct ==
  u1 : Inport  Port=1  PortWidth=-1  SampleTime=-1  DataType=auto
      settings: SignalType=auto
  u2 : Inport  Port=2  PortWidth=-1  SampleTime=-1  DataType=auto
      settings: SignalType=auto
  Demux : Demux  Outputs=3
  Demux1 : Demux  Outputs=3
  Mux1 : Mux  Inputs=3
  Sum : Sum  Inputs=+-  SaturateOnIntegerOverflow=on
  Sum1 : Sum  Inputs=-+  SaturateOnIntegerOverflow=on
  Sum2 : Sum  Inputs=+-  SaturateOnIntegerOverflow=on
  x1.y2 : Product  Inputs=2  SaturateOnIntegerOverflow=on
  x1.z2 : Product  Inputs=2  SaturateOnIntegerOverflow=on
  y1.x2 : Product  Inputs=2  SaturateOnIntegerOverflow=on
  y1.z2 : Product  Inputs=2  SaturateOnIntegerOverflow=on
  z1.x2 : Product  Inputs=2  SaturateOnIntegerOverflow=on
  z1.y2 : Product  Inputs=2  SaturateOnIntegerOverflow=on
  v : Outport  Port=1
  wires:
  u1/1 -> Demux1/1
  Demux1/2 -> y1.z2/1, y1.x2/1
  Demux1/1 -> x1.y2/1, x1.z2/1
  Demux1/3 -> z1.x2/1, z1.y2/1
  y1.z2/1 -> Sum/1
  z1.y2/1 -> Sum/2
  x1.z2/1 -> Sum1/1
  z1.x2/1 -> Sum1/2
  x1.y2/1 -> Sum2/1
  y1.x2/1 -> Sum2/2
  Sum1/1 -> Mux1/2
  Sum/1 -> Mux1/1
  Sum2/1 -> Mux1/3
  Mux1/1 -> v/1
  Demux/3 -> y1.z2/2, x1.z2/2
  Demux/2 -> x1.y2/2, z1.y2/2
  Demux/1 -> z1.x2/2, y1.x2/2
  u2/1 -> Demux/1
